simulink model "w2025b"  (R2025b)
settings: Solver=VariableStepAuto  StartTime=0.0  StopTime=60  RelTol=1e-3
values from neighbouring files (symbols this model uses):
  b1 = 0.008    [definicje.m]
  J = 0.03    [definicje.m]
  kf = 1.8/6.5    (= 0.276923076923)    [definicje.m]
  Ra = 3.0724    [definicje.m]
  tau = La/Ra    (= 0.0214334071084)    [definicje.m]
  Tl = 1    [definicje.m]
  Ua = 230    [definicje.m]
settings Model: Creator=Student  LastModifiedBy=Piotr
settings ModelReferenceCC: EnableRefExpFcnMdlSchedulingChecks=on
settings RTWCC: GPUComputeCapability=3.5
settings SimscapeCC: SimscapeLogDataHistory=5000  SimscapeLogDecimation=1

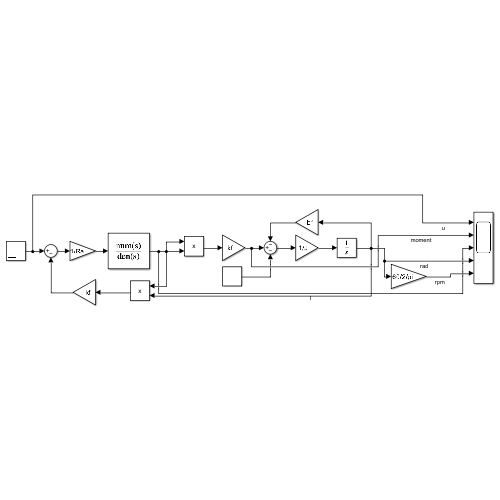
[thumbnail: Simulink's stored preview of the top-level diagram]
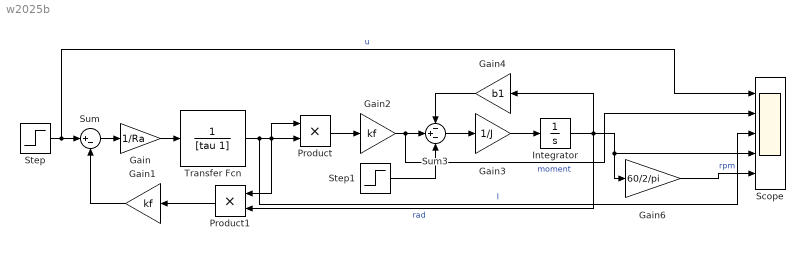
== system w2025b ==
  Gain : Gain  Gain=1/Ra
  Gain1 : Gain  Gain=kf
  Gain2 : Gain  Gain=kf
  Gain3 : Gain  Gain=1/J
  Gain4 : Gain  Gain=b1
  Gain6 : Gain  Gain=60/2/pi
  Integrator : Integrator
  Product : Product
  Product1 : Product
  Scope : Scope  NumInputPorts=5
      settings: ActiveDisplayYMinimum=-327.644922224124  ActiveDisplayYMaximum=2571.1599966613385
  Step : Step  After=Ua  SampleTime=0
  Step1 : Step  After=Tl  SampleTime=0
  Sum : Sum  Inputs=|+-
  Sum3 : Sum  Inputs=-+-
  Transfer Fcn : TransferFcn  Denominator=[tau 1]
  wires:
  Sum/1 -> Gain/1
  Gain/1 -> Transfer Fcn/1
  Gain2/1 -> Scope/2, Sum3/2  "moment"
  Sum3/1 -> Gain3/1
  Gain3/1 -> Integrator/1
  Integrator/1 -> Scope/4, Gain6/1, Gain4/1, Product1/2  "rad"
  Gain4/1 -> Sum3/1
  Step/1 -> Scope/1, Sum/1  "u"
  Product/1 -> Gain2/1
  Transfer Fcn/1 -> Scope/3, Product/2, Product1/1, Product/1  "I"
  Product1/1 -> Gain1/1
  Gain1/1 -> Sum/2
  Gain6/1 -> Scope/5  "rpm"
  Step1/1 -> Sum3/3
